simulink model "C_Dugoff_Tire_Model"  (R2022b)
settings: Solver=VariableStepAuto  StartTime=0.0  StopTime=10.0  RelTol=1e-3
values from neighbouring files (symbols this model uses):
  alpha = a_deg * pi/180    [complicated_dugoff.m]
  Cx = 50000    [complicated_dugoff.m]
  Cy = 30000    [complicated_dugoff.m]
  Fz = 3000    [complicated_dugoff.m]
  mu = 0.85    [complicated_dugoff.m]
  s = s_input    (= 0.1)    [complicated_dugoff.m]
settings Model: Creator=FATMANURATA  LastModifiedBy=FATMANURATA

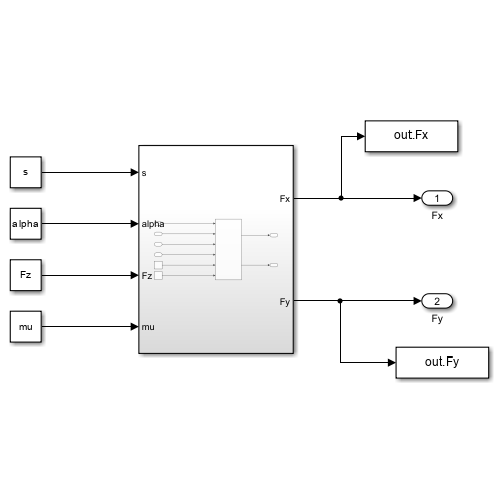
[thumbnail: Simulink's stored preview of the top-level diagram]
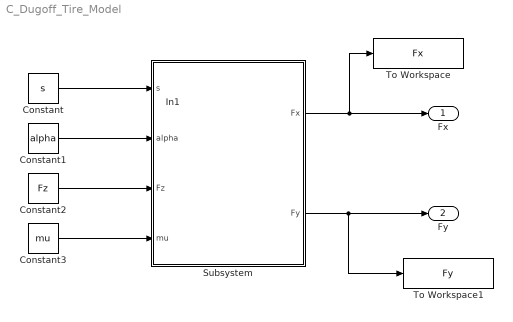
== system C_Dugoff_Tire_Model ==
  In1 : Inport
  Constant : Constant  Value=s
  Constant1 : Constant  Value=alpha
  Constant2 : Constant  Value=Fz
  Constant3 : Constant  Value=mu
  Subsystem : Subsystem
  To Workspace : ToWorkspace  VariableName=Fx  SampleTime=-1
  To Workspace1 : ToWorkspace  VariableName=Fy  SampleTime=-1
  Fx : Outport
  Fy : Outport  Port=2
  wires:
  Constant3/1 -> Subsystem/4(mu)
  Constant2/1 -> Subsystem/3(Fz)
  Constant1/1 -> Subsystem/2(alpha)
  Constant/1 -> Subsystem/1(s)
  Subsystem/1(Fx) -> Fx/1, To Workspace/1
  Subsystem/2(Fy) -> To Workspace1/1, Fy/1

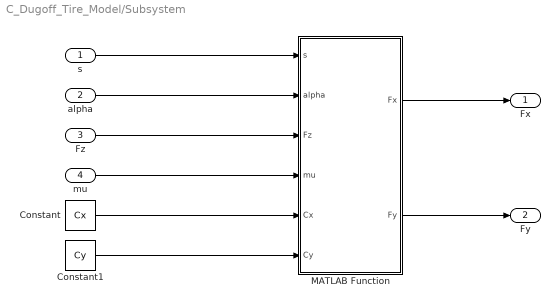
== system C_Dugoff_Tire_Model/Subsystem ==
  s : Inport
  alpha : Inport  Port=2
  Fz : Inport  Port=3
  mu : Inport  Port=4
  Constant : Constant  Value=Cx
  Constant1 : Constant  Value=Cy
  MATLAB Function : MATLAB Function  TreatAsAtomicUnit=on
  Fx : Outport
  Fy : Outport  Port=2
  wires:
  alpha/1 -> MATLAB Function/2(alpha)
  s/1 -> MATLAB Function/1(s)
  Fz/1 -> MATLAB Function/3(Fz)
  mu/1 -> MATLAB Function/4(mu)
  Constant/1 -> MATLAB Function/5(Cx)
  Constant1/1 -> MATLAB Function/6(Cy)
  MATLAB Function/1(Fx) -> Fx/1
  MATLAB Function/2(Fy) -> Fy/1

== matlab function C_Dugoff_Tire_Model/Subsystem/MATLAB Function ==
  data: s input; Fx output; alpha input; Fz input; mu input; Cx input; Cy input; Fy output
function [Fx, Fy] = fcn(s, alpha, Fz, mu, Cx, Cy)

    assert(isscalar(s));
    assert(isscalar(alpha));

    ta = tan(alpha);
    n = mu * Fz * (1 + s);
    dn = 2 * sqrt((Cx * s)^2 + (Cy * ta)^2);
    
    if dn == 0
        S = 100; % Bölme hatasını önlemek için büyük bir değer
    else
        S = n / dn;
    end

    % 2. f(S) fonksiyonu (Slayt 39 ortası)
    if S < 1
        fS = S * (2 - S);
    else
        fS = 1;
    end

    Fx = (Cx * s / (1 + s)) * fS;
    Fy = (Cy * ta / (1 + s)) * fS;
end
